simulink model "PMC"  (Simulink 6.5)
settings: Solver=ode45  StartTime=0.0  StopTime=10.0  RelTol=1e-3
undefined symbols (not defined in the file): pmctau2, pmctau3
settings Model: Creator=lfd  LastModifiedBy=lfd  ExtModeAutoUpdateStatusClock=off

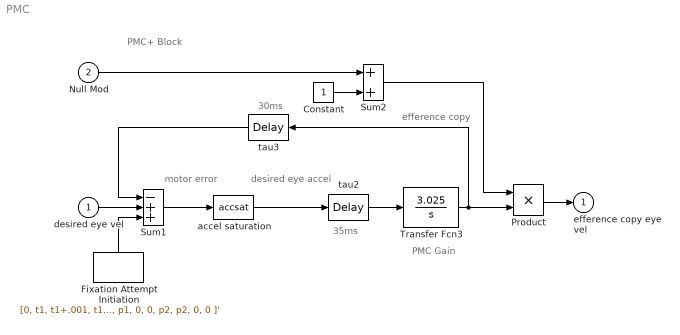
== system PMC ==
  note: desired
      | eye accel
  note: motor
      | error
  note: efference
      | copy
  note: PMC Gain
  note: 30ms
  note: 35ms
  note: PMC+ Block
  desired eye vel : Inport
  Null Mod : Inport  Port=2
  Constant : Constant
  Fixation Attempt Initiation : FromWorkspace  Orientation=up  VariableName=[0, t1, t1+.001, t1+d1, t1+d1+.001, t1+d1+.001+ipd, t1+d1+.001+ipd, t1+d1+.001+ipd+d2, t1+d1+.001+ipd+d2, 10000; 0, 0, p1, p1, 0, 0, p2, p2, 0, 0 ]'  mask{@1=825, @2=0, @3=.002, @4=.050, @5=-925, @6=.002}
      mask prompts: @1 "Pulse 1 Magnitude"; @2 "Time of Pulse 1 Onset"; @3 "Pulse 1 Duration"; @4 "Interpulse Delay"; @5 "Pulse 2 Magnitude"; @6 "Pulse 2 Duration"
      mask help: Double Pulse
      mask init:
      | p1=@1; t1=@2; d1=@3; ipd=@4; p2=@5; d2=@6;
      mask Display: disp('Double\nPulse')
  Product : Product  RndMeth=Zero
  Sum1 : Sum  Inputs=-++  SaturateOnIntegerOverflow=on  InputSameDT=on
  Sum2 : Sum  SaturateOnIntegerOverflow=on  InputSameDT=on
  Transfer Fcn3 : TransferFcn  Numerator=[3.025]  Denominator=[1 0]
  accel saturation : MATLABFcn  MATLABFcn=accsat
      mask Display: plot([-80 -4 4 80],[-120 -40 40 120], [0 0],[-120 120],[-80 80],[0 0])
  tau2 : TransportDelay  DelayTime=pmctau2/1000
  tau3 : TransportDelay  Orientation=left  DelayTime=pmctau3/1000
  efference copy eye vel : Outport  InitialOutput=0
  wires:
  accel saturation/1 -> tau2/1
  tau2/1 -> Transfer Fcn3/1
  Sum1/1 -> accel saturation/1
  tau3/1 -> Sum1/1
  desired eye vel/1 -> Sum1/2
  Transfer Fcn3/1 -> tau3/1, Product/2
  Fixation Attempt Initiation/1 -> Sum1/3
  Null Mod/1 -> Sum2/1
  Product/1 -> efference copy eye vel/1
  Sum2/1 -> Product/1
  Constant/1 -> Sum2/2
